simulink model "FSK"  (R2016a)
settings: Solver=FixedStepDiscrete  StartTime=0.0  StopTime=1.1  FixedStep=1/2000000  RelTol=1e-3
libraries: dsparch4 x5, dspsigops x1
settings Model: Creator=savt2301  LastModifiedBy=camj3302
settings SolverCC: AutoInsertRateTranBlk=on

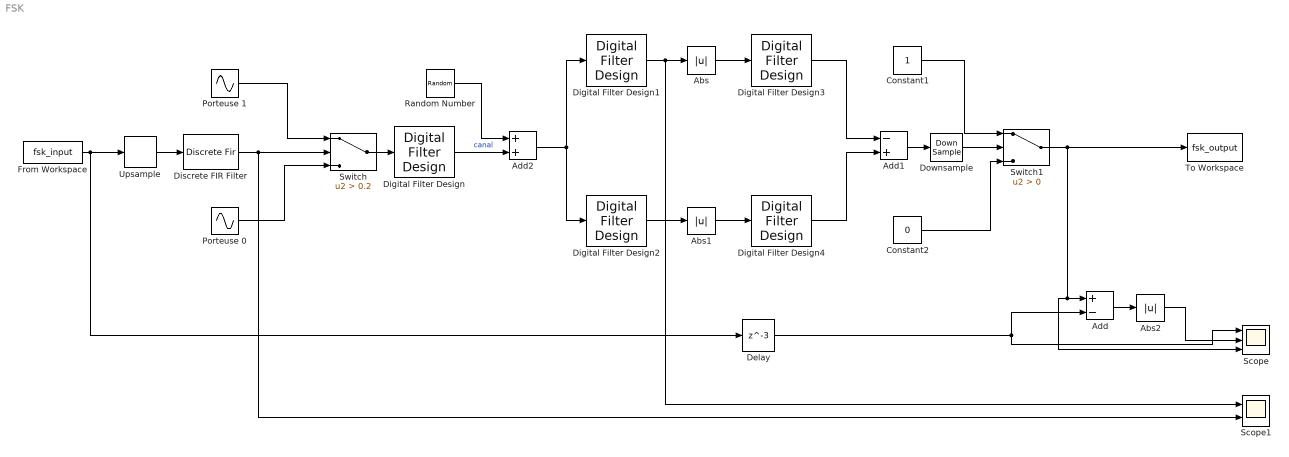
== system FSK ==
  Abs : Abs
  Abs1 : Abs
  Abs2 : Abs
  Add : Sum  Inputs=+-
  Add1 : Sum  Inputs=-+
  Add2 : Sum
  Constant1 : Constant  SampleTime=-1
  Constant2 : Constant  Value=0  SampleTime=-1
  Delay : Delay  DelayLength=3  InitialCondition=1
  Digital Filter Design{,1..4} (5 alike) : dsparch4/Digital Filter Design  mwdsp_browser_bugfix_var=off
  Discrete FIR Filter : DiscreteFir  Coefficients=ones(1,2000)
  Downsample : DownSample  N=2000  RateOptions=Allow multirate processing
  From Workspace : FromWorkspace  VariableName=fsk_input  SampleTime=1/1000
  Porteuse 0 : Sin  Frequency=72500*2*pi  SampleTime=1/2000000
  Porteuse 1 : Sin  Frequency=77500*2*pi  SampleTime=1/2000000
  Random Number : RandomNumber  Variance=20  SampleTime=1/2000000
  Scope : Scope  NumInputPorts=3
  Scope1 : Scope  NumInputPorts=2
  Switch : Switch  Criteria=u2 > Threshold  Threshold=0.2
  Switch1 : Switch  Criteria=u2 > Threshold
  To Workspace : ToWorkspace  VariableName=fsk_output  SampleTime=-1
      settings: Save2DSignal=2-D array (concatenate along first dimension)
  Upsample : dspsigops/Upsample  N=2000  phase=0  InputProcessing=Columns as channels (frame based)  RateOptions=Allow multirate processing  ic=0  mode=Unused parameter value
  wires:
  Porteuse 0/1 -> Switch/3
  Porteuse 1/1 -> Switch/1
  Digital Filter Design4/1 -> Add1/2
  Digital Filter Design3/1 -> Add1/1
  Digital Filter Design1/1 -> Scope1/1, Abs/1
  Abs/1 -> Digital Filter Design3/1
  Digital Filter Design2/1 -> Abs1/1
  Abs1/1 -> Digital Filter Design4/1
  Constant2/1 -> Switch1/3
  Constant1/1 -> Switch1/1
  Add/1 -> Abs2/1
  Abs2/1 -> Scope/2
  From Workspace/1 -> Upsample/1, Delay/1
  Switch1/1 -> To Workspace/1, Scope/3, Add/1
  Delay/1 -> Add/2, Scope/1
  Add1/1 -> Downsample/1
  Switch/1 -> Digital Filter Design/1
  Upsample/1 -> Discrete FIR Filter/1
  Discrete FIR Filter/1 -> Switch/2, Scope1/2
  Downsample/1 -> Switch1/2
  Digital Filter Design/1 -> Add2/2  "canal"
  Random Number/1 -> Add2/1
  Add2/1 -> Digital Filter Design2/1, Digital Filter Design1/1
